simulink model "qnd_random"  (R2021a)
settings: Solver=VariableStepAuto  StartTime=0.0  StopTime=100  RelTol=1e-3
PreLoadFcn:
  | preload_fcn
values from neighbouring files (symbols this model uses):
  BW = 10e3    (= 10000)    [preload_fcn.m]
  Fs = OSR*BW    (= 25600)    [preload_fcn.m]
  H = tf([1 0 (2*pi*1e3)^2],[1 2*pi*1e3 (2*pi*1e3)^2])    [preload_fcn.m]
  NFFT = 1024    [preload_fcn.m]
libraries: dsparch4 x1, dspsrcs4 x1
settings Model: Creator=kschutz  LastModifiedBy=kschutz

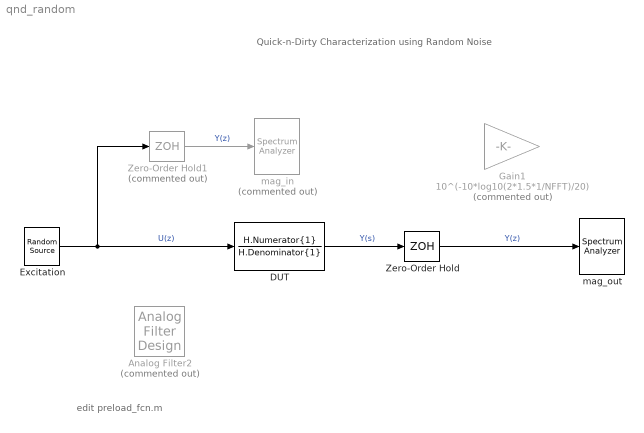
== system qnd_random ==
  note: edit preload_fcn.m
  note: Quick-n-Dirty Characterization
      | using Random Noise
  Analog Filter2 : dsparch4/Analog Filter Design  Commented=on  method=Elliptic  filttype=Lowpass  N=8  Wlo=2*pi*BW  Whi=80  Rp=.5  Rs=80
  DUT : TransferFcn  Numerator=H.Numerator{1}  Denominator=H.Denominator{1}
  Excitation : dspsrcs4/Random Source  SrcType=Gaussian  NormMethod=Ziggurat  CltLength=12  MinVal=0  MaxVal=1  MeanVal=0  VarVal=1  RepMode=Specify seed  rawSeed=123  IsInherit=off  SampMode=Discrete  SampTime=1/(Fs)  SampFrame=1  DataType=Double  OutComplex=Real  OutputFrames=off
  Gain1 : Gain  Commented=on  Gain=10^(-10*log10(2*1.5*1/NFFT)/20)
  Zero-Order Hold : ZeroOrderHold  SampleTime=1/(Fs)
  Zero-Order Hold1 : ZeroOrderHold  Commented=on  SampleTime=1/(10*Fs)
  mag_in : SpectrumAnalyzer  Commented=on
  mag_out : SpectrumAnalyzer
  wires:
  Zero-Order Hold/1 -> mag_out/1  "Y(z)"
  Excitation/1 -> DUT/1, Zero-Order Hold1/1  "U(z)"
  Zero-Order Hold1/1 -> mag_in/1  "Y(z)"
  DUT/1 -> Zero-Order Hold/1  "Y(s)"
